simulink model "hastighet"  (R2014b)
settings: Solver=ode45  StartTime=0.0  StopTime=10  RelTol=1e-3
values from neighbouring files (symbols this model uses):
  k = 100    [eulers_metode_d.m]    (also in eulers_metode_og_ekakt.m; pitch_main.m; sim_system.m)
  m = 200    [eulers_metode_d.m]    (also in eulers_metode_og_ekakt.m; pitch_main.m; sim_system.m)
  v_0 = 0    [pitch_main.m]    (also in sim_system.m)
settings Model: Creator=rende_000  LastModifiedBy=rende_000

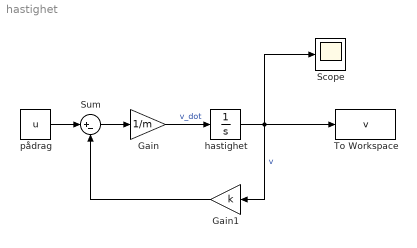
== system hastighet ==
  Gain : Gain  Gain=1/m
  Gain1 : Gain  Gain=k
  Scope : Scope
      settings: TimeRange=15  YMin=0
  Sum : Sum  Inputs=|+-
  To Workspace : ToWorkspace  VariableName=v  SaveFormat=Timeseries  SampleTime=-1
  hastighet : Integrator  InitialCondition=v_0
  pådrag : Constant  Value=u
  wires:
  hastighet/1 -> To Workspace/1, Gain1/1, Scope/1  "v"
  Sum/1 -> Gain/1
  Gain/1 -> hastighet/1  "v_dot"
  pådrag/1 -> Sum/1
  Gain1/1 -> Sum/2
